simulink model "Syr_ctrl_SFun"  (R2020b)
settings: Solver=ode45  StartTime=0.0  StopTime=4  FixedStep=Tstep  MaxStep=Tstep  RelTol=1e-3  AbsTol=1e-3  EnableMultiTasking=on
InitFcn:
  | tic
  | init_sim
  | mex Syr_ctrl.c User_functions\Src\*.c
StopFcn:
  | elapsed_time=toc
values from neighbouring files (symbols this model uses):
  accel = 5000    [init_sim.m]
  Bm = 0.    (= 0)    [init_sim.m]
  Clarke = 2/3*[1 -0.5 -0.5;0 sqrt(3)/2 -sqrt(3)/2]    [init_sim.m]
  Clarke_inv = [1 0;-0.5 sqrt(3)/2;-0.5 -sqrt(3)/2]    [init_sim.m]
  Ctrl_type = 3    [init_sim.m]
  dem = 1    [init_sim.m]
  dT = motorModel.SyreDrive.Converter.dT * 1e-6    [init_sim.m]
  F0_alpha = Fd0*cos(th0) - Fq0*sin(th0)    [init_sim.m]
  F0_beta = Fd0*sin(th0) + Fq0*cos(th0)    [init_sim.m]
  Fd = motorModel.FluxMapInv_dq.Fd    [init_sim.m]
  Fd_max = max(motorModel.FluxMapInv_dqt.dataF.Fd,[],'all')    [init_sim.m]
  Fd_min = min(motorModel.FluxMapInv_dqt.dataF.Fd,[],'all')    [init_sim.m]
  FMapsModel = -1    [init_sim.m]
  Fq = motorModel.FluxMapInv_dq.Fq    [init_sim.m]
  Fq_max = max(motorModel.FluxMapInv_dqt.dataF.Fq,[],'all')    [init_sim.m]
  Fq_min = min(motorModel.FluxMapInv_dqt.dataF.Fq,[],'all')    [init_sim.m]
  HS_ctrl = 1    [init_sim.m]
  Id_dqt = interpn(motorModel.FluxMapInv_dqt.dataF.Fd,motorModel.FluxMapInv_dqt.dataF.Fq,motorModel.FluxMapInv_dqt.dataF.th,motorModel.FluxMapInv_dqt.dataF.Id,Fd_dqt,Fq_dqt,th_dqt,'cubic')    [init_sim.m]
  id_MTPA = interp1(abs(MTPA.id+1i*MTPA.iq),MTPA.id,i0)    [init_sim.m]
  inj_waveform = 1    [init_sim.m]
  Iq_dqt = interpn(motorModel.FluxMapInv_dqt.dataF.Fd,motorModel.FluxMapInv_dqt.dataF.Fq,motorModel.FluxMapInv_dqt.dataF.th,motorModel.FluxMapInv_dqt.dataF.Iq,Fd_dqt,Fq_dqt,th_dqt,'cubic')    [init_sim.m]
  iq_MTPA = interp1(abs(MTPA.id+1i*MTPA.iq),MTPA.iq,i0)    [init_sim.m]
  J = motorModel.data.J    [init_sim.m]
  p = motorModel.data.p    [init_sim.m]
  Quad_Maps = 2    [init_sim.m]
  Rd = motorModel.SyreDrive.Converter.Rd    [init_sim.m]
  Rfe = 1e5    (= 100000)    [init_sim.m]
  Rs = motorModel.data.Rs    [init_sim.m]
  SS_on = 1    [init_sim.m]
  T_dqt = interpn(motorModel.FluxMapInv_dqt.dataF.Fd,motorModel.FluxMapInv_dqt.dataF.Fq,motorModel.FluxMapInv_dqt.dataF.th,motorModel.FluxMapInv_dqt.dataF.T,Fd_dqt,Fq_dqt,th_dqt,'cubic')    [init_sim.m]
  Tf = 0    [init_sim.m]
  th0 = 0    [init_sim.m]
  th_max = max(motorModel.FluxMapInv_dqt.dataF.th,[],'all')    [init_sim.m]
  th_min = min(motorModel.FluxMapInv_dqt.dataF.th,[],'all')    [init_sim.m]
  Ts = 100e-6    (= 0.0001)    [init_sim.m]
  Tv = 0    [init_sim.m]
  VDC = motorModel.data.Vdc    [init_sim.m]
undefined symbols (not defined in the file or in its folder): magnitude, sigbuilder_block, T0
settings Model: SimulationMode=accelerator  Creator=work  LastModifiedBy=Ananth
settings SolverCC: AutoScaleAbsTol=off
settings DataIOCC: FinalStateName=xFinalSim  InitialState=xFinalSim  SaveFormat=Array  SignalLoggingSaveFormat=ModelDataLogs  SaveOutput=off  SignalLogging=off  DSMLogging=off  TimeSaveName=time  SignalLoggingName=sigsOut
settings OptimizationCC: BlockReduction=off  BooleanDataType=off  ExpressionDepthLimit=2147483647  InitFltsAndDblsToZero=on  LifeSpan=inf
settings DebuggingCC: SaveWithParameterizedLinksMsg=none  UnderspecifiedInitializationDetection=Classic  MergeDetectMultiDrivingBlocksExec=none  SignalResolutionControl=TryResolveAllWithWarning  MultiTaskDSMMsg=warning  MultiTaskCondExecSysMsg=none  FcnCallInpInsideContextMsg=warning  StateNameClashWarn=warning  SFUnexpectedBacktrackingDiag=warning  SFNoUnconditionalDefaultTransitionDiag=warning  SFExecutionAtInitializationDiag=none  ArithmeticOperatorsInVariantConditions=warning
settings HardwareCC: ProdBitPerPointer=32  ProdBitPerSizeT=32  ProdBitPerPtrDiffT=32  ProdLargestAtomicFloat=None  ProdIntDivRoundTo=Undefined  ProdEndianess=Unspecified  ProdWordSize=32  ProdHWDeviceType=32-bit Generic  TargetBitPerPointer=64  TargetBitPerSizeT=64  TargetBitPerPtrDiffT=64  TargetLongLongMode=on  TargetIntDivRoundTo=Zero  TargetEndianess=LittleEndian  TargetWordSize=64  TargetHWDeviceType=MATLAB Host  ProdEqTarget=off
settings ModelReferenceCC: PropagateSignalLabelsOutOfModel=off
settings SFSimCC: SimUseLocalCustomCode=off  CustomCodeUndefinedFunction=UseInterfaceOnly
settings RTWCC: RTWUseLocalCustomCode=off
settings CodeAppCC: StateflowObjectComments=on
settings GRTTargetCC: TargetFcnLib=ansi_tfl_tmw.mat  TargetLangStandard=C89/C90 (ANSI)  CombineOutputUpdateFcns=off  GRTInterface=on
settings ConfigComp: CovMetricSettings=dw  CovSaveCumulativeToWorkspaceVar=on  CovSaveSingleToWorkspaceVar=on  CovExternalEMLEnable=off  CovSFcnEnable=off

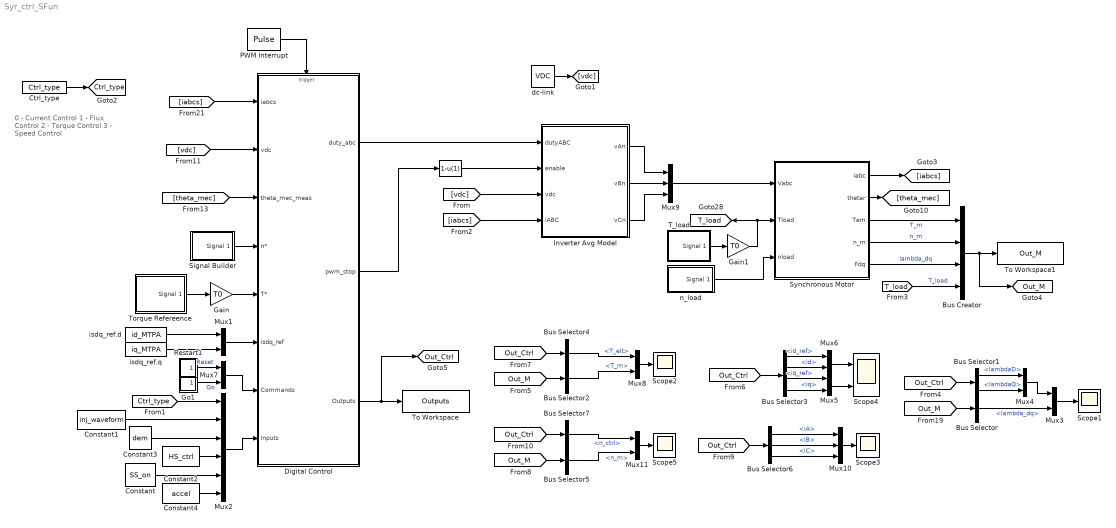
== system Syr_ctrl_SFun ==
  note: 0 - Current Control
      | 1 - Flux Control
      | 2 - Torque Control
      | 3 - Speed Control
  " " : Fcn  Expr=1-u(1)
  Bus Creator : BusCreator  Inputs=4
  Bus Selector : BusSelector  OutputSignals=lambda_dq
  Bus Selector1 : BusSelector  OutputSignals=lambdaD,lambdaQ
  Bus Selector2 : BusSelector  OutputSignals=T_m
  Bus Selector3 : BusSelector  OutputSignals=id_ref,id,iq_ref,iq
  Bus Selector4 : BusSelector  OutputSignals=T_elt
  Bus Selector5 : BusSelector  OutputSignals=n_m
  Bus Selector6 : BusSelector  OutputSignals=iA,iB,iC
  Bus Selector7 : BusSelector  OutputSignals=n_ctrl
  Constant : Constant  Value=SS_on
  Constant1 : Constant  Value=inj_waveform
  Constant2 : Constant  Value=HS_ctrl
  Constant3 : Constant  Value=dem
  Constant4 : Constant  Value=accel
  Ctrl_type : Constant  Value=Ctrl_type
  Digital Control : Subsystem  TreatAsAtomicUnit=on
  Gain : Gain  Gain=T0
  Gain1 : Gain  Gain=T0
  Go1 : Subsystem
  Inverter Avg Model : Subsystem  mask{TR_mdl=2 Parameters (Von; Rd), TR_par=[0 Rd 3 1.5 0.0714], D_mdl=2 Parameters (Vf; Rd), D_par=[0 Rd 3 0 0], fsw=1/Ts*1e-3, dead_time=dT*1e6, enable_dt=on, enable_vdrop=on}
      mask prompts: TR_mdl "Choose Transistor model"; TR_par "Transistor parameters [Von1 (V), Rd1 (ohm), Iknee (A), Von2 (V), Rd2 (ohm)]"; D_mdl "Choose Diode model"; D_par "Diode parameters [Vf1 (V), Rd1 (ohm), Iknee (A), Vf2 (V), Rd2 (ohm)]"; fsw "Switching frequency (kHz)"; dead_time "Inverter dead-time (microseconds)"; enable_dt "Enable dead-time effects"; enable_vdrop "Enable on-state voltage drops"
      mask help:
      | This averaged model represents a generic inverter. Select the type of components model to calculate the voltage drop and then insert the parameters value.
      | The requested parameters must be inserted as [von1, Rd1, Iknee, von2 Rd2]. If "2 Parameters" is selected Iknee, von2 and Rd2 are neglected. Iknee is the current at which the voltage drop model passes from (von1, Rd1) to (von2, Rd2).
      mask TypeOptions TR_mdl: 2 Parameters (Von; Rd) | 5 Parameters (Von1; Rd1; Iknee; Von2; Rd2)
      mask TypeOptions D_mdl: 2 Parameters (Vf; Rd) | 5 Parameters (Vf1; Rd1; Iknee; Vf2; Rd2)
      mask Display: plot(0,0,100,100,[39 39 23.8],[71 28 28],[44 56 49.6 56 52.8 56 61 61],[39.2 33.6 32.8 33.6 40.8 33.6 30 12.4],[44 44 44 61 61],[28 71 60 66.4 90],[75 67 83 75 67 83 75 75],[54 42 42 54 54 54 54 66],[61 75 75],[24 24 42],[75 75 61],[66,76,76]);
  Mux{1,3..8,11} (8 alike) : Mux  Inputs=2
  Mux10 : Mux  Inputs=3
  Mux2 : Mux  Inputs=6
  Mux9 : Mux  Inputs=3
  PWM Interrupt : DiscretePulseGenerator  PulseType=Time based  Period=Ts  PulseWidth=50
  Restart1 : Subsystem
  Scope{1..3,5} (4 alike) : Scope
  Scope4 : Scope  NumInputPorts=2
  Signal Builder : Subsystem  Tag=STV Subsys  LoadFcn=sigbuilder_block('load');  StartFcn=sigbuilder_block('start');  StopFcn=sigbuilder_block('stop');  ClipboardFcn=sigbuilder_block('clipboard');  mask(Sigbuilder block){tuvar=[0:10]}
      mask help: Simulink:masks:SigbuilderBlock_MD
      mask init:
      | if ~strcmp(get_param(bdroot(gcbh),'SimulationStatus'),'stopped') tuvar = sigbuilder_block('maskInit'); end
      settings: CopyFcn=sigbuilder_block('copy');  DeleteFcn=sigbuilder_block('delete');  ModelCloseFcn=sigbuilder_block('modelClose');  PreSaveFcn=sigbuilder_block('preSave');  PauseFcn=sigbuilder_block('pause');  ContinueFcn=sigbuilder_block('continue');  NameChangeFcn=sigbuilder_block('namechange');  OpenFcn=sigbuilder_block('open',[312 77.4 550.2 399.6 ]);  CloseFcn=sigbuilder_block('close');
      mask Display: plot(0, 0, 100, 100,[2, 2, 32, 32, 2], [68, 8, 8, 68, 68],[32, 2], [38, 38], [32, 19, 2],[53, 60, 44], [32, 17, 17, 2],[16, 16, 31, 31]);txt = getActiveGroup(gcbh);text(2, 100, txt,'verticalAlignment', 'top');
  Synchronous Motor : Subsystem
      mask init:
      | %init_ind_motor_sat;
      | %if (flag_pfe==0)
      | %	Rfe=inf;
      | %end
      | %if (flag_pfe==0)
      | %	Rfe=inf;
      | %end
      mask Display: disp('Motor Model');
  T_load : Subsystem  Tag=STV Subsys  LoadFcn=sigbuilder_block('load');  StartFcn=sigbuilder_block('start');  StopFcn=sigbuilder_block('stop');  ClipboardFcn=sigbuilder_block('clipboard');  mask(Sigbuilder block){tuvar=[0:10]}
      mask help: Simulink:masks:SigbuilderBlock_MD
      mask init:
      | if ~strcmp(get_param(bdroot(gcbh),'SimulationStatus'),'stopped') tuvar = sigbuilder_block('maskInit'); end
      settings: CopyFcn=sigbuilder_block('copy');  DeleteFcn=sigbuilder_block('delete');  ModelCloseFcn=sigbuilder_block('modelClose');  PreSaveFcn=sigbuilder_block('preSave');  PauseFcn=sigbuilder_block('pause');  ContinueFcn=sigbuilder_block('continue');  NameChangeFcn=sigbuilder_block('namechange');  OpenFcn=sigbuilder_block('open',[537 153.6 550.2 360.6 ]);  CloseFcn=sigbuilder_block('close');
      mask Display: plot(0, 0, 100, 100,[2, 2, 32, 32, 2], [68, 8, 8, 68, 68],[32, 2], [38, 38], [32, 19, 2],[53, 60, 44], [32, 17, 17, 2],[16, 16, 31, 31]);txt = getActiveGroup(gcbh);text(2, 100, txt,'verticalAlignment', 'top');
  To Workspace : ToWorkspace  VariableName=Outputs  SaveFormat=Timeseries  SampleTime=-1
  To Workspace1 : ToWorkspace  VariableName=Out_M  SaveFormat=Timeseries  SampleTime=-1
  Torque Refereence : Subsystem  Tag=STV Subsys  LoadFcn=sigbuilder_block('load');  StartFcn=sigbuilder_block('start');  StopFcn=sigbuilder_block('stop');  ClipboardFcn=sigbuilder_block('clipboard');  mask(Sigbuilder block){tuvar=[0:10]}
      mask help: Simulink:masks:SigbuilderBlock_MD
      mask init:
      | if ~strcmp(get_param(bdroot(gcbh),'SimulationStatus'),'stopped') tuvar = sigbuilder_block('maskInit'); end
      settings: CopyFcn=sigbuilder_block('copy');  DeleteFcn=sigbuilder_block('delete');  ModelCloseFcn=sigbuilder_block('modelClose');  PreSaveFcn=sigbuilder_block('preSave');  PauseFcn=sigbuilder_block('pause');  ContinueFcn=sigbuilder_block('continue');  NameChangeFcn=sigbuilder_block('namechange');  OpenFcn=sigbuilder_block('open',[454.2 151.2 550.2 360.6 ]);  CloseFcn=sigbuilder_block('close');
      mask Display: plot(0, 0, 100, 100,[2, 2, 32, 32, 2], [68, 8, 8, 68, 68],[32, 2], [38, 38], [32, 19, 2],[53, 60, 44], [32, 17, 17, 2],[16, 16, 31, 31]);txt = getActiveGroup(gcbh);text(2, 100, txt,'verticalAlignment', 'top');
  dc-link : Constant  Value=VDC
  isdq_ref.d : Constant  Value=id_MTPA
  isdq_ref.q : Constant  Value=iq_MTPA
  n_load : Subsystem  Tag=STV Subsys  LoadFcn=sigbuilder_block('load');  StartFcn=sigbuilder_block('start');  StopFcn=sigbuilder_block('stop');  ClipboardFcn=sigbuilder_block('clipboard');  mask(Sigbuilder block){tuvar=[0:10]}
      mask help: Simulink:masks:SigbuilderBlock_MD
      mask init:
      | if ~strcmp(get_param(bdroot(gcbh),'SimulationStatus'),'stopped') tuvar = sigbuilder_block('maskInit'); end
      settings: CopyFcn=sigbuilder_block('copy');  DeleteFcn=sigbuilder_block('delete');  ModelCloseFcn=sigbuilder_block('modelClose');  PreSaveFcn=sigbuilder_block('preSave');  PauseFcn=sigbuilder_block('pause');  ContinueFcn=sigbuilder_block('continue');  NameChangeFcn=sigbuilder_block('namechange');  OpenFcn=sigbuilder_block('open',[46.8 30.6 550.2 354.6 ]);  CloseFcn=sigbuilder_block('close');
      mask Display: plot(0, 0, 100, 100,[2, 2, 32, 32, 2], [68, 8, 8, 68, 68],[32, 2], [38, 38], [32, 19, 2],[53, 60, 44], [32, 17, 17, 2],[16, 16, 31, 31]);txt = getActiveGroup(gcbh);text(2, 100, txt,'verticalAlignment', 'top');
  tag scope: Ctrl_type=global, Out_Ctrl=global, Out_M=global, T_load=global
  wires:
  dc-link/1 -> [vdc]
  Digital Control/1(duty_abc) -> Inverter Avg Model/1(dutyABC)
  Digital Control/2(pwm_stop) -> " "/1
  [iabcs] -> Digital Control/1(iabcs)
  [vdc] -> Digital Control/2(vdc)
  Mux7/1 -> Digital Control/7(Commands)
  " "/1 -> Inverter Avg Model/2(enable)
  PWM Interrupt/1 -> Digital Control/Trigger
  Restart1/1(Res) -> Mux7/1  "Reset"
  Go1/1(Go) -> Mux7/2  "Go"
  Synchronous Motor/2(thetar) -> [theta_mec]
  Synchronous Motor/1(iabc) -> [iabcs]
  Mux9/1 -> Synchronous Motor/1(Vabc)
  Gain1/1 -> Synchronous Motor/2(Tload), [T_load]
  Inverter Avg Model/1(vAn) -> Mux9/1
  Inverter Avg Model/2(vBn) -> Mux9/2
  Inverter Avg Model/3(vCn) -> Mux9/3
  [vdc] -> Inverter Avg Model/3(vdc)
  Mux1/1 -> Digital Control/6(isdq_ref)
  isdq_ref.d/1 -> Mux1/1
  isdq_ref.q/1 -> Mux1/2
  Ctrl_type/1 -> [Ctrl_type]
  n_load/1(Signal 1) -> Synchronous Motor/3(nload)
  Gain/1 -> Digital Control/5(T*)
  [theta_mec] -> Digital Control/3(theta_mec_meas)
  [Ctrl_type] -> Mux2/1
  Constant1/1 -> Mux2/2
  Constant3/1 -> Mux2/3
  Constant2/1 -> Mux2/4
  Mux2/1 -> Digital Control/8(Inputs)
  Signal Builder/1(Signal 1) -> Digital Control/4(n*)
  Constant/1 -> Mux2/5
  T_load/1(Signal 1) -> Gain1/1
  Digital Control/3(Outputs) -> [Out_Ctrl], To Workspace/1
  Torque Refereence/1(Signal 1) -> Gain/1
  Synchronous Motor/3(Tem) -> Bus Creator/1  "T_m"
  Synchronous Motor/4(n_m) -> Bus Creator/2  "n_m"
  Synchronous Motor/5(Fdq) -> Bus Creator/3  "lambda_dq"
  Bus Creator/1 -> To Workspace1/1, [Out_M]
  [T_load] -> Bus Creator/4  "T_load"
  Constant4/1 -> Mux2/6
  Mux3/1 -> Scope1/1
  [Out_M] -> Bus Selector/1
  [Out_Ctrl] -> Bus Selector1/1
  Bus Selector1/1 -> Mux4/1  "<lambdaD>"
  Bus Selector1/2 -> Mux4/2  "<lambdaQ>"
  Bus Selector/1 -> Mux3/2  "<lambda_dq>"
  Mux4/1 -> Mux3/1
  Bus Selector3/2 -> Mux6/2  "<id>"
  Bus Selector3/1 -> Mux6/1  "<id_ref>"
  [Out_Ctrl] -> Bus Selector3/1
  Mux6/1 -> Scope4/1
  Mux5/1 -> Scope4/2
  Bus Selector3/3 -> Mux5/1  "<iq_ref>"
  Bus Selector3/4 -> Mux5/2  "<iq>"
  Bus Selector2/1 -> Mux8/2  "<T_m>"
  Bus Selector4/1 -> Mux8/1  "<T_elt>"
  [Out_Ctrl] -> Bus Selector4/1
  [Out_M] -> Bus Selector2/1
  Mux8/1 -> Scope2/1
  Mux10/1 -> Scope3/1
  [Out_Ctrl] -> Bus Selector6/1
  Bus Selector6/1 -> Mux10/1  "<iA>"
  Bus Selector6/2 -> Mux10/2  "<iB>"
  Bus Selector6/3 -> Mux10/3  "<iC>"
  Mux11/1 -> Scope5/1
  [Out_M] -> Bus Selector5/1
  [Out_Ctrl] -> Bus Selector7/1
  Bus Selector7/1 -> Mux11/1  "<n_ctrl>"
  Bus Selector5/1 -> Mux11/2  "<n_m>"
  [iabcs] -> Inverter Avg Model/4(iABC)

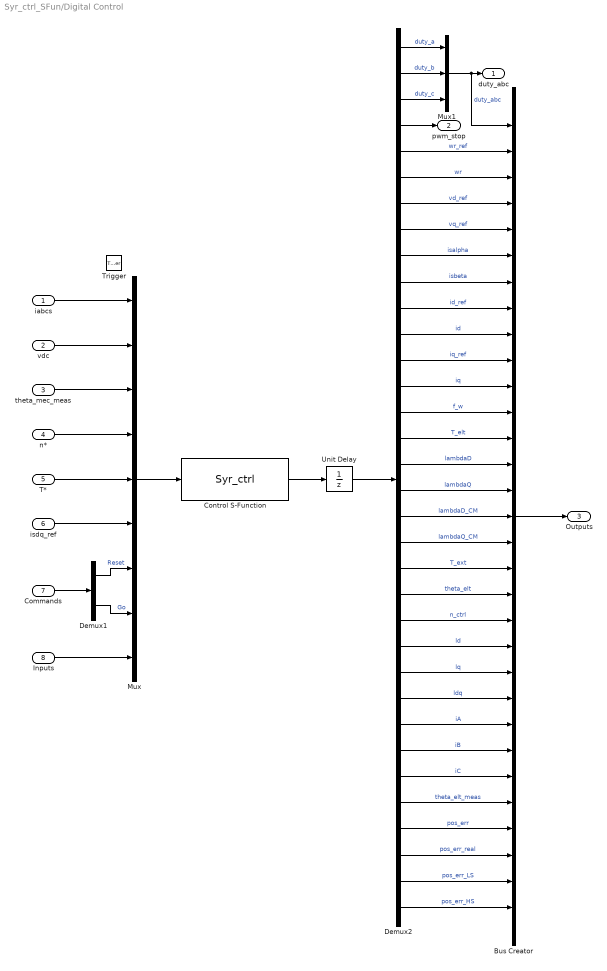
== system Syr_ctrl_SFun/Digital Control ==
  iabcs : Inport
  vdc : Inport  Port=2
  theta_mec_meas : Inport  Port=3
  n* : Inport  Port=4
  T* : Inport  Port=5
  isdq_ref : Inport  Port=6
  Commands : Inport  Port=7
  Inputs : Inport  Port=8
  Trigger : TriggerPort  VariantControl=(inherit)
  Bus Creator : BusCreator  Inputs=31
  Control S-Function : S-Function  FunctionName=Syr_ctrl  SFunctionDeploymentMode=off  EnableBusSupport=off
  Demux1 : Demux  Outputs=2
  Demux2 : Demux  Outputs=34
  Mux : Mux  Inputs=9
  Mux1 : Mux  Inputs=3
  Unit Delay : UnitDelay  SampleTime=-1  HasFrameUpgradeWarning=on
  duty_abc : Outport
  pwm_stop : Outport  Port=2
  Outputs : Outport  Port=3
  wires:
  Mux/1 -> Control S-Function/1
  iabcs/1 -> Mux/1
  vdc/1 -> Mux/2
  theta_mec_meas/1 -> Mux/3
  Control S-Function/1 -> Unit Delay/1
  n*/1 -> Mux/4
  Mux1/1 -> Bus Creator/1, duty_abc/1  "duty_abc"
  Demux1/1 -> Mux/7  "Reset"
  Demux1/2 -> Mux/8  "Go"
  Commands/1 -> Demux1/1
  isdq_ref/1 -> Mux/6
  Unit Delay/1 -> Demux2/1
  Demux2/1 -> Mux1/1  "duty_a"
  Demux2/2 -> Mux1/2  "duty_b"
  Demux2/3 -> Mux1/3  "duty_c"
  Demux2/4 -> pwm_stop/1
  T*/1 -> Mux/5
  Inputs/1 -> Mux/9
  Bus Creator/1 -> Outputs/1
  Demux2/34 -> Bus Creator/31  "pos_err_HS"
  Demux2/33 -> Bus Creator/30  "pos_err_LS"
  Demux2/32 -> Bus Creator/29  "pos_err_real"
  Demux2/31 -> Bus Creator/28  "pos_err"
  Demux2/30 -> Bus Creator/27  "theta_elt_meas"
  Demux2/29 -> Bus Creator/26  "iC"
  Demux2/28 -> Bus Creator/25  "iB"
  Demux2/27 -> Bus Creator/24  "iA"
  Demux2/26 -> Bus Creator/23  "ldq"
  Demux2/25 -> Bus Creator/22  "lq"
  Demux2/24 -> Bus Creator/21  "ld"
  Demux2/23 -> Bus Creator/20  "n_ctrl"
  Demux2/22 -> Bus Creator/19  "theta_elt"
  Demux2/21 -> Bus Creator/18  "T_ext"
  Demux2/20 -> Bus Creator/17  "lambdaQ_CM"
  Demux2/18 -> Bus Creator/15  "lambdaQ"
  Demux2/19 -> Bus Creator/16  "lambdaD_CM"
  Demux2/17 -> Bus Creator/14  "lambdaD"
  Demux2/16 -> Bus Creator/13  "T_elt"
  Demux2/15 -> Bus Creator/12  "f_w"
  Demux2/14 -> Bus Creator/11  "iq"
  Demux2/13 -> Bus Creator/10  "iq_ref"
  Demux2/12 -> Bus Creator/9  "id"
  Demux2/11 -> Bus Creator/8  "id_ref"
  Demux2/10 -> Bus Creator/7  "isbeta"
  Demux2/9 -> Bus Creator/6  "isalpha"
  Demux2/8 -> Bus Creator/5  "vq_ref"
  Demux2/7 -> Bus Creator/4  "vd_ref"
  Demux2/6 -> Bus Creator/3  "wr"
  Demux2/5 -> Bus Creator/2  "wr_ref"

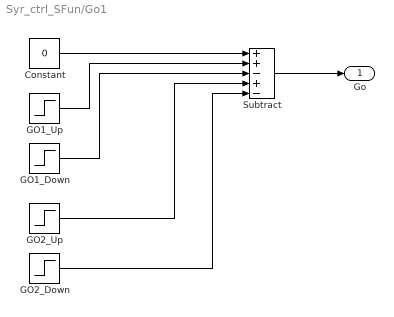
== system Syr_ctrl_SFun/Go1 ==
  Constant : Constant  Value=0
  GO1_Down : Step  Time=0.03+4*Ts  SampleTime=0
  GO1_Up : Step  Time=0.03  SampleTime=0
  GO2_Down : Step  Time=0.1+4*Ts  SampleTime=0
  GO2_Up : Step  Time=0.1  SampleTime=0
  Subtract : Sum  Inputs=++-+-
  Go : Outport
  wires:
  Subtract/1 -> Go/1
  Constant/1 -> Subtract/1
  GO1_Up/1 -> Subtract/2
  GO1_Down/1 -> Subtract/3
  GO2_Up/1 -> Subtract/4
  GO2_Down/1 -> Subtract/5

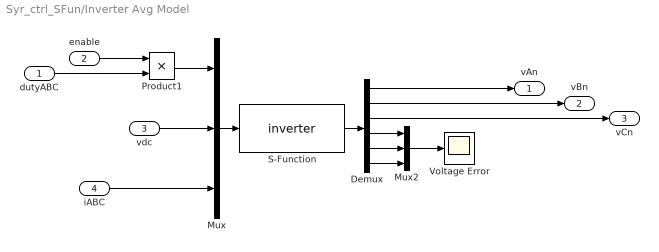
== system Syr_ctrl_SFun/Inverter Avg Model ==
  dutyABC : Inport
  enable : Inport  Port=2
  vdc : Inport  Port=3
  iABC : Inport  Port=4
  Demux : Demux  Outputs=6
      settings: DisplayOption=none
  Mux : Mux  Inputs=3
  Mux2 : Mux  Inputs=3
  Product1 : Product  RndMeth=Zero
  S-Function : S-Function  FunctionName=inverter  Parameters=fsw,dead_time,enable_dt,enable_vdrop, TR_par(1), TR_par(2), TR_par(3), TR_par(4), TR_par(5), D_par(1), D_par(2), D_par(3), D_par(4), D_par(5), TR_mdl, D_mdl  SFunctionDeploymentMode=off  EnableBusSupport=off
  Voltage Error : Scope
  vAn : Outport  VectorParamsAs1DForOutWhenUnconnected=off
  vBn : Outport  Port=2  VectorParamsAs1DForOutWhenUnconnected=off
  vCn : Outport  Port=3  VectorParamsAs1DForOutWhenUnconnected=off
  wires:
  Demux/6 -> Mux2/3
  Demux/5 -> Mux2/2
  Demux/4 -> Mux2/1
  dutyABC/1 -> Product1/2
  Product1/1 -> Mux/1
  Demux/3 -> vCn/1
  Demux/2 -> vBn/1
  Demux/1 -> vAn/1
  vdc/1 -> Mux/2
  Mux/1 -> S-Function/1
  S-Function/1 -> Demux/1
  enable/1 -> Product1/1
  Mux2/1 -> Voltage Error/1
  iABC/1 -> Mux/3

== system Syr_ctrl_SFun/Restart1 ==
  "DOWN " : Step  Time=10e-3+4*Ts  SampleTime=0
  Subtract : Sum  Inputs=+-
  "UP " : Step  Time=10e-3  SampleTime=0
  Res : Outport
  wires:
  "UP "/1 -> Subtract/1
  "DOWN "/1 -> Subtract/2
  Subtract/1 -> Res/1

== system Syr_ctrl_SFun/Signal Builder ==
  Demux : Demux  Tag=STV Demux  Outputs=1
      settings: DisplayOption=none
  FromWs : FromWorkspace  Tag=STV FromWs  VariableName=tuvar
      SigBuilderData=|
      | common.afterFinalStr = 'Extrapolate'
      | common.sampleTime = 0
      | dataSet.timeRange = [0 10]
      | dataSet.name = 'Group 1'
      | sbobj.Groups.Name = 'Group 1'
      | sbobj.Groups.Signals.Name = 'Signal 1'
      | sbobj.Groups.Signals.XData = [0 1.98 1.98 8 8 10]
      | sbobj.Groups.Signals.YData = [0 0 1500 1500 -1500 -1500]
  Signal 1 : Outport  Tag=STV Outport
  wires:
  Demux/1 -> Signal 1/1
  FromWs/1 -> Demux/1

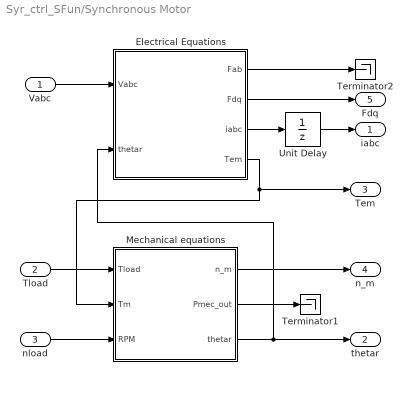
== system Syr_ctrl_SFun/Synchronous Motor ==
  Vabc : Inport
  Tload : Inport  Port=2
  nload : Inport  Port=3
  Electrical Equations : Subsystem
  Mechanical equations : Subsystem
  Terminator1 : Terminator
  Terminator2 : Terminator
  Unit Delay : UnitDelay  SampleTime=-1  HasFrameUpgradeWarning=on
  iabc : Outport
  thetar : Outport  Port=2
  Tem : Outport  Port=3
  n_m : Outport  Port=4
  Fdq : Outport  Port=5
  wires:
  Mechanical equations/3(thetar) -> Electrical Equations/2(thetar), thetar/1
  Electrical Equations/4(Tem) -> Tem/1, Mechanical equations/2(Tm)
  Electrical Equations/2(Fdq) -> Fdq/1
  Electrical Equations/3(iabc) -> Unit Delay/1
  Electrical Equations/1(Fab) -> Terminator2/1
  Mechanical equations/2(Pmec_out) -> Terminator1/1
  Mechanical equations/1(n_m) -> n_m/1
  Tload/1 -> Mechanical equations/1(Tload)
  Unit Delay/1 -> iabc/1
  Vabc/1 -> Electrical Equations/1(Vabc)
  nload/1 -> Mechanical equations/3(RPM)

== system Syr_ctrl_SFun/T_load ==
  Demux : Demux  Tag=STV Demux  Outputs=1
      settings: DisplayOption=none
  FromWs : FromWorkspace  Tag=STV FromWs  VariableName=tuvar
      SigBuilderData=|
      | common.afterFinalStr = 'Extrapolate'
      | common.sampleTime = 0
      | dataSet.timeRange = [0 10]
      | dataSet.name = 'Group 1'
      | sbobj.Groups.Name = 'Group 1'
      | sbobj.Groups.Signals.Name = 'Signal 1'
      | sbobj.Groups.Signals.XData = [0 0.5 0.5 1.02 1.02 8.64 8.64 10]
      | sbobj.Groups.Signals.YData = [0 0 -0.5 -0.5 0.5 0.5 -0.98 -0.98]
  Signal 1 : Outport  Tag=STV Outport
  wires:
  FromWs/1 -> Demux/1
  Demux/1 -> Signal 1/1

== system Syr_ctrl_SFun/Torque Refereence ==
  Demux : Demux  Tag=STV Demux  Outputs=1
      settings: DisplayOption=none
  FromWs : FromWorkspace  Tag=STV FromWs  VariableName=tuvar
      SigBuilderData=|
      | common.afterFinalStr = 'Extrapolate'
      | common.sampleTime = 0
      | dataSet.timeRange = [0 10]
      | dataSet.name = 'Group 1'
      | sbobj.Groups.Name = 'Group 1'
      | sbobj.Groups.Signals.Name = 'Signal 1'
      | sbobj.Groups.Signals.XData = [0 0.56 0.56 3 3 5.14 5.14 10]
      | sbobj.Groups.Signals.YData = [0 0 1 1 -1 -1 0 0]
  Signal 1 : Outport  Tag=STV Outport
  wires:
  FromWs/1 -> Demux/1
  Demux/1 -> Signal 1/1

== system Syr_ctrl_SFun/n_load ==
  Demux : Demux  Tag=STV Demux  Outputs=1
      settings: DisplayOption=none
  FromWs : FromWorkspace  Tag=STV FromWs  VariableName=tuvar
      SigBuilderData=|
      | common.afterFinalStr = 'Extrapolate'
      | common.sampleTime = 0
      | dataSet.timeRange = [0 10]
      | dataSet.name = 'Group 1'
      | sbobj.Groups.Name = 'Group 1'
      | sbobj.Groups.Signals.Name = 'Signal 1'
      | sbobj.Groups.Signals.XData = [0 0.98 2.48 6.72 6.72 10]
      | sbobj.Groups.Signals.YData = [0 0 1000 1000 5 5]
  Signal 1 : Outport  Tag=STV Outport
  wires:
  Demux/1 -> Signal 1/1
  FromWs/1 -> Demux/1

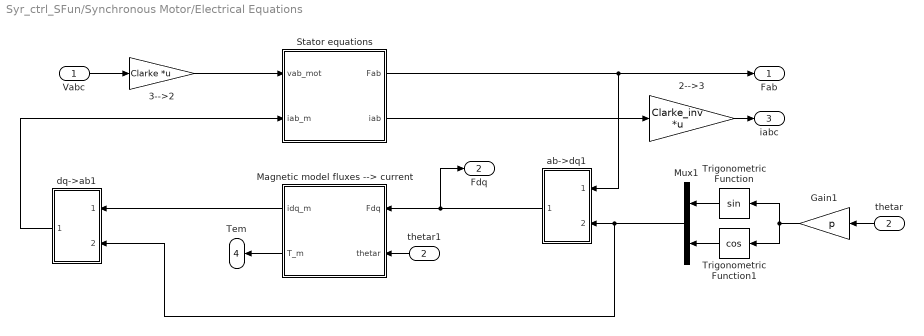
== system Syr_ctrl_SFun/Synchronous Motor/Electrical Equations ==
  Vabc : Inport
  thetar : Inport  Port=2
  2-->3 : Gain  Gain=Clarke_inv  Multiplication=Matrix(K*u)  SaturateOnIntegerOverflow=on  OutDataTypeStr=Inherit: Same as input  ParamDataTypeStr=Inherit: Same as input
  3-->2 : Gain  Gain=Clarke  Multiplication=Matrix(K*u)  SaturateOnIntegerOverflow=on  OutDataTypeStr=Inherit: Same as input  ParamDataTypeStr=Inherit: Same as input
  Gain1 : Gain  Gain=p  SaturateOnIntegerOverflow=on  OutDataTypeStr=Inherit: Same as input  ParamDataTypeStr=Inherit: Same as input
  Magnetic model fluxes --> current : Subsystem
  Mux1 : Mux  Inputs=2
  Stator equations : Subsystem
  Trigonometric Function : Trigonometry
  Trigonometric Function1 : Trigonometry  Operator=cos
  ab->dq1 : Subsystem
      mask Display: disp('A(-theta)')
  dq->ab1 : Subsystem
      mask Display: disp('A(theta)')
  thetar1 : InportShadow  Port=2
  Fab : Outport
  Fdq : Outport  Port=2
  iabc : Outport  Port=3
  Tem : Outport  Port=4
  wires:
  3-->2/1 -> Stator equations/1(vab_mot)
  Stator equations/1(Fab) -> ab->dq1/1(X_ab), Fab/1
  ab->dq1/1(X_dq) -> Fdq/1, Magnetic model fluxes --> current/1(Fdq)
  Vabc/1 -> 3-->2/1
  Stator equations/2(iab) -> 2-->3/1
  2-->3/1 -> iabc/1
  Mux1/1 -> dq->ab1/2(sin,cos), ab->dq1/2(sin,cos)
  dq->ab1/1(X_dq) -> Stator equations/2(iab_m)
  Magnetic model fluxes --> current/1(idq_m) -> dq->ab1/1(X_ab)
  Magnetic model fluxes --> current/2(T_m) -> Tem/1
  Trigonometric Function/1 -> Mux1/1
  Trigonometric Function1/1 -> Mux1/2
  Gain1/1 -> Trigonometric Function/1, Trigonometric Function1/1
  thetar/1 -> Gain1/1
  thetar1/1 -> Magnetic model fluxes --> current/2(thetar)

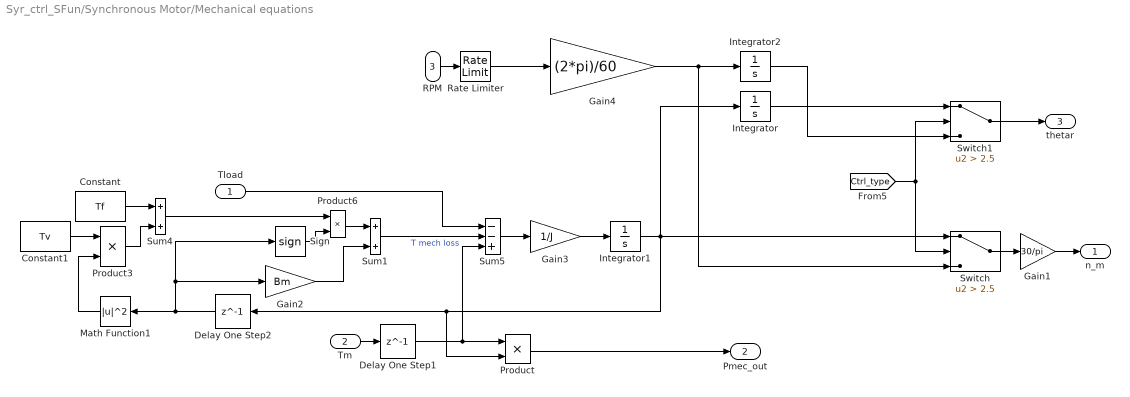
== system Syr_ctrl_SFun/Synchronous Motor/Mechanical equations ==
  Tload : Inport
  Tm : Inport  Port=2
  RPM : Inport  Port=3
  Constant : Constant  Value=Tf
  Constant1 : Constant  Value=Tv
  Delay One Step1 : Delay  DelayLength=1
  Delay One Step2 : Delay  DelayLength=1
  Gain1 : Gain  Gain=30/pi
  Gain2 : Gain  Gain=Bm  SaturateOnIntegerOverflow=on  OutDataTypeStr=Inherit: Same as input  ParamDataTypeStr=Inherit: Same as input
  Gain3 : Gain  Gain=1/J  SaturateOnIntegerOverflow=on  OutDataTypeStr=Inherit: Same as input  ParamDataTypeStr=Inherit: Same as input
  Gain4 : Gain  Gain=(2*pi)/60
  Integrator : Integrator  InitialCondition=th0  WrapState=on  WrappedStateUpperValue=2*pi  WrappedStateLowerValue=0
  Integrator1 : Integrator
  Integrator2 : Integrator  InitialCondition=th0  WrapState=on  WrappedStateUpperValue=2*pi  WrappedStateLowerValue=0
  Math Function1 : Math  Operator=magnitude^2  SignedPower=on  SaturateOnIntegerOverflow=on
  Product : Product  SaturateOnIntegerOverflow=on  OutDataTypeStr=Inherit: Same as first input
  Product3 : Product  SaturateOnIntegerOverflow=on  OutDataTypeStr=Inherit: Same as first input
  Product6 : Product  SaturateOnIntegerOverflow=on  OutDataTypeStr=Inherit: Same as first input
  Rate Limiter : RateLimiter  RisingSlewLimit=accel  FallingSlewLimit=-accel  SampleTimeMode=inherited
  Sign : Signum  ZeroCross=off
  Sum1 : Sum  SaturateOnIntegerOverflow=on  OutDataTypeStr=Inherit: Same as first input
  Sum4 : Sum  SaturateOnIntegerOverflow=on  OutDataTypeStr=Inherit: Same as first input
  Sum5 : Sum  Inputs=--+  SaturateOnIntegerOverflow=on  OutDataTypeStr=Inherit: Same as first input
  Switch : Switch  Criteria=u2 > Threshold  Threshold=2.5
  Switch1 : Switch  Criteria=u2 > Threshold  Threshold=2.5
  n_m : Outport
  Pmec_out : Outport  Port=2  VectorParamsAs1DForOutWhenUnconnected=off
  thetar : Outport  Port=3
  wires:
  Gain3/1 -> Integrator1/1
  Gain2/1 -> Sum1/2
  Delay One Step2/1 -> Math Function1/1, Sign/1, Gain2/1
  Product6/1 -> Sum1/1
  Sum1/1 -> Sum5/2  "T mech loss"
  Tm/1 -> Delay One Step1/1
  Product/1 -> Pmec_out/1
  Tload/1 -> Sum5/1
  Math Function1/1 -> Product3/2
  Constant1/1 -> Product3/1
  Product3/1 -> Sum4/2
  Constant/1 -> Sum4/1
  Sum5/1 -> Gain3/1
  Sign/1 -> Product6/2
  Sum4/1 -> Product6/1
  Integrator2/1 -> Switch1/3
  Integrator/1 -> Switch1/1
  Switch1/1 -> thetar/1
  Switch/1 -> Gain1/1
  Integrator1/1 -> Integrator/1, Switch/1, Delay One Step2/1, Product/2
  Gain4/1 -> Switch/3, Integrator2/1
  [Ctrl_type] -> Switch/2, Switch1/2
  RPM/1 -> Rate Limiter/1
  Rate Limiter/1 -> Gain4/1
  Delay One Step1/1 -> Sum5/3, Product/1
  Gain1/1 -> n_m/1

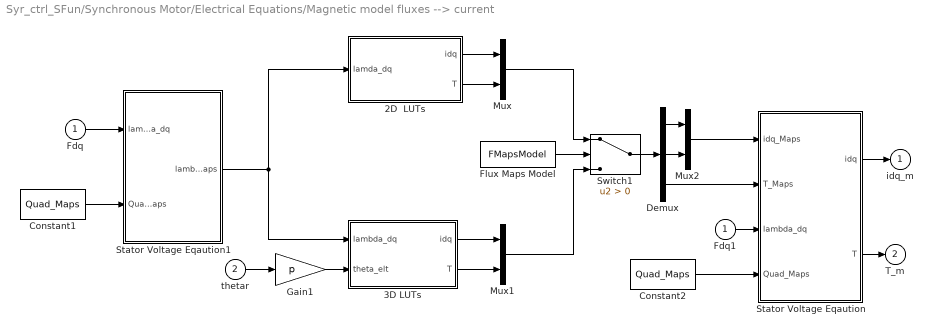
== system Syr_ctrl_SFun/Synchronous Motor/Electrical Equations/Magnetic model fluxes --> current ==
  Fdq : Inport
  thetar : Inport  Port=2
  2D  LUTs : Subsystem
  3D LUTs : Subsystem
  Constant1 : Constant  Value=Quad_Maps
  Constant2 : Constant  Value=Quad_Maps
  Demux : Demux  Outputs=3
  Fdq1 : InportShadow
  Flux Maps Model : Constant  Value=FMapsModel
  Gain1 : Gain  Gain=p  SaturateOnIntegerOverflow=on  OutDataTypeStr=Inherit: Same as input  ParamDataTypeStr=Inherit: Same as input
  Mux : Mux  Inputs=2
  Mux1 : Mux  Inputs=2
  Mux2 : Mux  Inputs=2
  Stator Voltage Eqaution : MATLAB Function  TreatAsAtomicUnit=on
  Stator Voltage Eqaution1 : MATLAB Function  TreatAsAtomicUnit=on
  Switch1 : Switch  Criteria=u2 > Threshold
  idq_m : Outport  InitialOutput=0
  T_m : Outport  Port=2  InitialOutput=0
  wires:
  Fdq/1 -> Stator Voltage Eqaution1/1(lambda_dq)
  Constant1/1 -> Stator Voltage Eqaution1/2(Quad_Maps)
  Fdq1/1 -> Stator Voltage Eqaution/3(lambda_dq)
  Constant2/1 -> Stator Voltage Eqaution/4(Quad_Maps)
  Stator Voltage Eqaution/1(idq) -> idq_m/1
  Flux Maps Model/1 -> Switch1/2
  Stator Voltage Eqaution1/1(lambda_dq_Maps) -> 3D LUTs/1(lambda_dq), 2D  LUTs/1(lamda_dq)
  Switch1/1 -> Demux/1
  thetar/1 -> Gain1/1
  Gain1/1 -> 3D LUTs/2(theta_elt)
  Stator Voltage Eqaution/2(T) -> T_m/1
  2D  LUTs/1(idq) -> Mux/1
  2D  LUTs/2(T) -> Mux/2
  3D LUTs/1(idq) -> Mux1/1
  3D LUTs/2(T) -> Mux1/2
  Mux/1 -> Switch1/1
  Mux1/1 -> Switch1/3
  Demux/1 -> Mux2/1
  Demux/2 -> Mux2/2
  Mux2/1 -> Stator Voltage Eqaution/1(idq_Maps)
  Demux/3 -> Stator Voltage Eqaution/2(T_Maps)

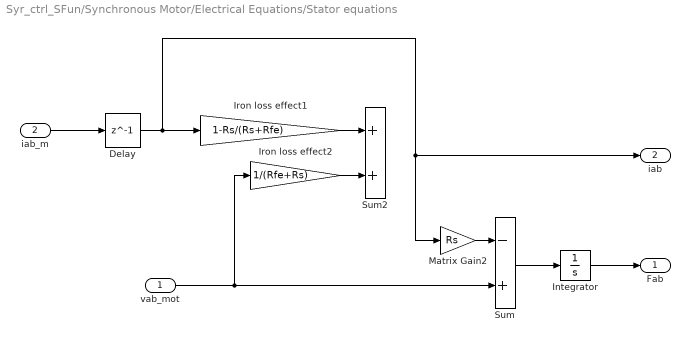
== system Syr_ctrl_SFun/Synchronous Motor/Electrical Equations/Stator equations ==
  vab_mot : Inport
  iab_m : Inport  Port=2
  Delay : Delay  DelayLength=1
  Integrator : Integrator  InitialCondition=[F0_alpha,F0_beta]
  Iron loss effect1 : Gain  Gain=1-Rs/(Rs+Rfe)  SaturateOnIntegerOverflow=on  OutDataTypeStr=Inherit: Same as input  ParamDataTypeStr=Inherit: Same as input
  Iron loss effect2 : Gain  Gain=1/(Rfe+Rs)  SaturateOnIntegerOverflow=on  OutDataTypeStr=Inherit: Same as input  ParamDataTypeStr=Inherit: Same as input
  Matrix Gain2 : Gain  Gain=Rs  SaturateOnIntegerOverflow=on  OutDataTypeStr=Inherit: Same as input  ParamDataTypeStr=Inherit: Same as input
  Sum : Sum  Inputs=-+  SaturateOnIntegerOverflow=on  OutDataTypeStr=Inherit: Same as first input
  Sum2 : Sum  SaturateOnIntegerOverflow=on  OutDataTypeStr=Inherit: Same as first input
  Fab : Outport  VectorParamsAs1DForOutWhenUnconnected=off
  iab : Outport  Port=2  VectorParamsAs1DForOutWhenUnconnected=off
  wires:
  Matrix Gain2/1 -> Sum/1
  iab_m/1 -> Delay/1
  vab_mot/1 -> Iron loss effect2/1, Sum/2
  Delay/1 -> iab/1, Matrix Gain2/1, Iron loss effect1/1
  Iron loss effect1/1 -> Sum2/1
  Iron loss effect2/1 -> Sum2/2
  Integrator/1 -> Fab/1
  Sum/1 -> Integrator/1

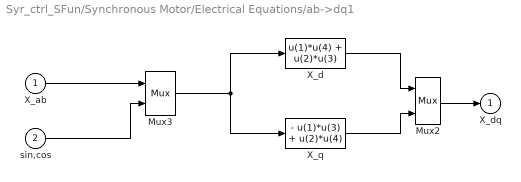
== system Syr_ctrl_SFun/Synchronous Motor/Electrical Equations/ab->dq1 ==
  X_ab : Inport
  sin,cos : Inport  Port=2
  Mux2 : Mux  Inputs=2
  Mux3 : Mux  Inputs=2
  X_d : Fcn  Expr=u(1)*u(4) + u(2)*u(3)
  X_q : Fcn  Expr=- u(1)*u(3) + u(2)*u(4)
  X_dq : Outport  InitialOutput=0
  wires:
  X_q/1 -> Mux2/2
  X_d/1 -> Mux2/1
  Mux3/1 -> X_q/1, X_d/1
  sin,cos/1 -> Mux3/2
  X_ab/1 -> Mux3/1
  Mux2/1 -> X_dq/1

== system Syr_ctrl_SFun/Synchronous Motor/Electrical Equations/dq->ab1 ==
  X_ab : Inport
  sin,cos : Inport  Port=2
  Mux2 : Mux  Inputs=2
  Mux3 : Mux  Inputs=2
  X_d1 : Fcn  Expr=u(1)*u(4) - u(2)*u(3)
  X_q1 : Fcn  Expr=u(1)*u(3) + u(2)*u(4)
  X_dq : Outport  InitialOutput=0
  wires:
  Mux2/1 -> X_dq/1
  X_ab/1 -> Mux3/1
  sin,cos/1 -> Mux3/2
  Mux3/1 -> X_d1/1, X_q1/1
  X_d1/1 -> Mux2/1
  X_q1/1 -> Mux2/2

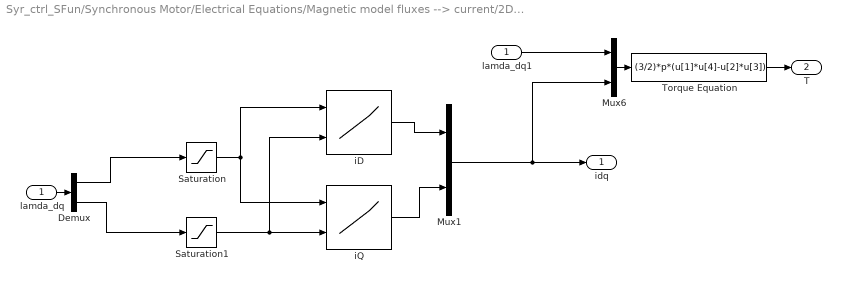
== system Syr_ctrl_SFun/Synchronous Motor/Electrical Equations/Magnetic model fluxes --> current/2D  LUTs ==
  lamda_dq : Inport
  Demux : Demux  Outputs=2
  Mux1 : Mux  Inputs=2
  Mux6 : Mux  Inputs=2
  Saturation : Saturate  UpperLimit=max(max(Fd))  LowerLimit=min(min(Fd))  LinearizeAsGain=off
  Saturation1 : Saturate  UpperLimit=max(max(Fq))  LowerLimit=min(min(Fq))  LinearizeAsGain=off
  Torque Equation : Fcn  Expr=(3/2)*p*(u[1]*u[4]-u[2]*u[3])
  iD : Lookup_n-D  BreakpointsForDimension1=Fd(1,:)  BreakpointsForDimension2=Fq(:,1)  BreakpointsForDimension1FirstPoint=0  BreakpointsForDimension2FirstPoint=0  BreakpointsForDimension1Spacing=0.17  BreakpointsForDimension2Spacing=0.17  Table=Id'  InternalRulePriority=Speed  RndMeth=Simplest  InputSameDT=on
      settings: InputPortMap=u0,u1
  iQ : Lookup_n-D  BreakpointsForDimension1=Fd(1,:)  BreakpointsForDimension2=Fq(:,1)  BreakpointsForDimension1FirstPoint=0  BreakpointsForDimension2FirstPoint=0  BreakpointsForDimension1Spacing=0.17  BreakpointsForDimension2Spacing=0.17  Table=Iq'  InternalRulePriority=Speed  RndMeth=Simplest  InputSameDT=on
      settings: InputPortMap=u0,u1
  lamda_dq1 : InportShadow
  idq : Outport
  T : Outport  Port=2
  wires:
  Demux/2 -> Saturation1/1
  Demux/1 -> Saturation/1
  Saturation/1 -> iD/1, iQ/1
  lamda_dq/1 -> Demux/1
  Saturation1/1 -> iD/2, iQ/2
  iD/1 -> Mux1/1
  iQ/1 -> Mux1/2
  lamda_dq1/1 -> Mux6/1
  Mux6/1 -> Torque Equation/1
  Mux1/1 -> Mux6/2, idq/1
  Torque Equation/1 -> T/1

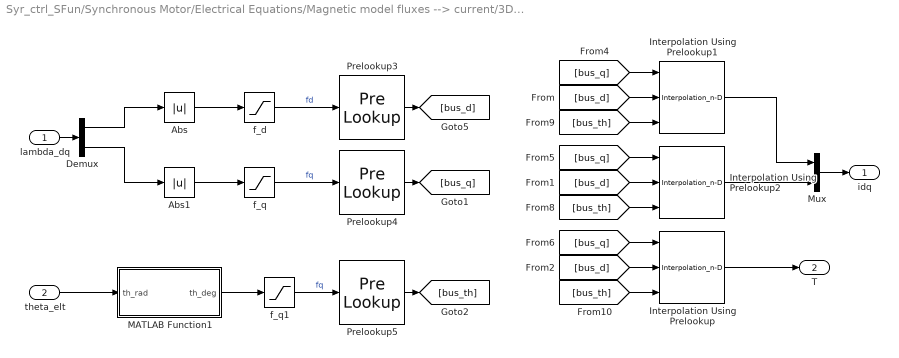
== system Syr_ctrl_SFun/Synchronous Motor/Electrical Equations/Magnetic model fluxes --> current/3D LUTs ==
  lambda_dq : Inport
  theta_elt : Inport  Port=2
  Abs : Abs
  Abs1 : Abs
  Demux : Demux  Outputs=2
  Interpolation Using Prelookup : Interpolation_n-D  NumberOfTableDimensions=3  Table=T_dqt  LookupTableObject=T_th  RequireIndexFractionAsBus=on  InternalRulePriority=Speed
      settings: InputPortMap=u0,u1,u2
  Interpolation Using Prelookup1 : Interpolation_n-D  NumberOfTableDimensions=3  Table=Id_dqt  RequireIndexFractionAsBus=on  InternalRulePriority=Speed
      settings: InputPortMap=u0,u1,u2
  Interpolation Using Prelookup2 : Interpolation_n-D  NumberOfTableDimensions=3  Table=Iq_dqt  RequireIndexFractionAsBus=on  InternalRulePriority=Speed
      settings: InputPortMap=u0,u1,u2
  MATLAB Function1 : MATLAB Function  TreatAsAtomicUnit=on
  Mux : Mux  Inputs=2
  Prelookup3 : PreLookup  BreakpointsData=Fd_v  OutputSelection=Index and fraction as bus  ExtrapMethod=Linear
  Prelookup4 : PreLookup  BreakpointsData=Fq_v  OutputSelection=Index and fraction as bus  ExtrapMethod=Linear
  Prelookup5 : PreLookup  BreakpointsData=th_v  OutputSelection=Index and fraction as bus  ExtrapMethod=Linear
  f_d : Saturate  UpperLimit=Fd_max  LowerLimit=Fd_min
  f_q : Saturate  UpperLimit=Fq_max  LowerLimit=Fq_min
  f_q1 : Saturate  UpperLimit=th_max  LowerLimit=th_min  ZeroCross=off
  idq : Outport
  T : Outport  Port=2
  wires:
  f_q1/1 -> Prelookup5/1  "fq"
  [bus_th] -> Interpolation Using Prelookup/3
  [bus_th] -> Interpolation Using Prelookup1/3
  [bus_th] -> Interpolation Using Prelookup2/3
  Prelookup5/1 -> [bus_th]
  [bus_q] -> Interpolation Using Prelookup/1
  [bus_q] -> Interpolation Using Prelookup2/1
  [bus_q] -> Interpolation Using Prelookup1/1
  Prelookup4/1 -> [bus_q]
  [bus_d] -> Interpolation Using Prelookup/2
  [bus_d] -> Interpolation Using Prelookup2/2
  [bus_d] -> Interpolation Using Prelookup1/2
  Prelookup3/1 -> [bus_d]
  Demux/2 -> Abs1/1
  Demux/1 -> Abs/1
  Interpolation Using Prelookup/1 -> T/1
  Abs1/1 -> f_q/1
  theta_elt/1 -> MATLAB Function1/1(th_rad)
  MATLAB Function1/1(th_deg) -> f_q1/1
  f_q/1 -> Prelookup4/1  "fq"
  f_d/1 -> Prelookup3/1  "fd"
  Mux/1 -> idq/1
  lambda_dq/1 -> Demux/1
  Abs/1 -> f_d/1
  Interpolation Using Prelookup1/1 -> Mux/1
  Interpolation Using Prelookup2/1 -> Mux/2

== matlab function Syr_ctrl_SFun/Synchronous Motor/Electrical Equations/Magnetic model fluxes --> current/Stator Voltage Eqaution ==
  data: idq_Maps input; T_Maps input; lambda_dq input; Quad_Maps input; idq output; T output
function [idq, T] = fcn(idq_Maps, T_Maps, lambda_dq, Quad_Maps)

idq = [0; 0];
T = 0;

if Quad_Maps == 0 %SyR
    idq(1) = idq_Maps(1)*sign(lambda_dq(1));
    idq(2) = idq_Maps(2)*sign(lambda_dq(2));
    T = T_Maps*sign(lambda_dq(1))*sign(lambda_dq(2));
end

if Quad_Maps == 1 %PM-SyR
    idq(1) = idq_Maps(1)*sign(lambda_dq(1));
    T = T_Maps*sign(lambda_dq(1));
end

if Quad_Maps == 2 %IPM
    idq(2) = idq_Maps(2)*sign(lambda_dq(2));
    T = T_Maps*sign(lambda_dq(2));
end

== matlab function Syr_ctrl_SFun/Synchronous Motor/Electrical Equations/Magnetic model fluxes --> current/Stator Voltage Eqaution1 ==
  data: lambda_dq input; Quad_Maps input; lambda_dq_Maps output
function lambda_dq_Maps = fcn(lambda_dq, Quad_Maps)

lambda_dq_Maps = [0; 0];
if Quad_Maps == 0 %SyR
    lambda_dq_Maps(1) = abs(lambda_dq(1));
    lambda_dq_Maps(2) = abs(lambda_dq(2));
end

if Quad_Maps == 1 %PM-SyR
    lambda_dq_Maps(1) = abs(lambda_dq(1));
end

if Quad_Maps == 2 %IPM
    lambda_dq_Maps(2) = abs(lambda_dq(2));
end

== matlab function Syr_ctrl_SFun/Synchronous Motor/Electrical Equations/Magnetic model fluxes --> current/3D LUTs/MATLAB Function1 ==
  data: th_rad input; th_deg output
function th_deg = fcn(th_rad)

th_deg=th_rad*180/pi;

while th_deg>360
    th_deg=th_deg-360;
end

while th_deg<0
    th_deg=th_deg+360;
end
